simulink model "carsim_experiment_validate"  (R2017a)
settings: Solver=VariableStepAuto  StartTime=0.0  StopTime=200  RelTol=1e-3
InitFcn:
  | set_param("carsim_experiment_validate/lk_system", ...
  | "Parameters",...
  | "[lk_acc_state.y.Data(1); lk_acc_state.nu.Data(1); lk_acc_state.dPsi.Data(1); lk_acc_state.r.Data(1)]")
undefined symbols (not defined in the file or in its folder): lk_acc_state
settings Model: Creator=User  LastModifiedBy=User

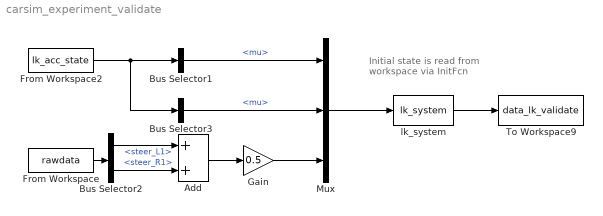
== system carsim_experiment_validate ==
  note: Initial state is read from workspace via InitFcn
  Add : Sum
  Bus Selector1 : BusSelector  OutputSignals=mu
  Bus Selector2 : BusSelector  OutputSignals=steer_L1,steer_R1
  Bus Selector3 : BusSelector  OutputSignals=mu
  From Workspace : FromWorkspace  VariableName=rawdata  OutDataTypeStr=Bus: DataBus  SampleTime=0
  From Workspace2 : FromWorkspace  VariableName=lk_acc_state  OutDataTypeStr=Bus: LKACCBus  SampleTime=0
  Gain : Gain  Gain=0.5
  Mux : Mux  Inputs=3
  To Workspace9 : ToWorkspace  VariableName=data_lk_validate  SaveFormat=Timeseries  SampleTime=-1
  lk_system : S-Function  FunctionName=lk_system  Parameters=[lk_acc_state.y.Data(1); lk_acc_state.nu.Data(1); lk_acc_state.dPsi.Data(1); lk_acc_state.r.Data(1)]  SFunctionDeploymentMode=off  EnableBusSupport=off
  wires:
  Mux/1 -> lk_system/1
  lk_system/1 -> To Workspace9/1
  From Workspace/1 -> Bus Selector2/1
  Bus Selector3/1 -> Mux/2  "<mu>"
  From Workspace2/1 -> Bus Selector3/1, Bus Selector1/1
  Bus Selector1/1 -> Mux/1  "<mu>"
  Bus Selector2/2 -> Add/2  "<steer_R1>"
  Bus Selector2/1 -> Add/1  "<steer_L1>"
  Gain/1 -> Mux/3
  Add/1 -> Gain/1
